simulink model "lab06es02_e1"  (R2021a)
settings: Solver=VariableStepAuto  StartTime=0.0  StopTime=150  RelTol=1e-3
values from neighbouring files (symbols this model uses):
  Kc = Kr/(Kf*0.2)    [L_11_05_21_reti_anticipatrici.m]    (also in L_11_05_21_reti_anticipatrici_2.m; L_12_05_21_Esercizio_progetto_di_un_controllore.m = 1/(0.04*Kf1*Kf2); L_12_05_21_effetti_sul_comando.m = 4; L_12_05_21_reti_integro-derivative.m = 4)
  Kr = 1    [L_11_05_21_reti_anticipatrici.m]    (also in L_11_05_21_reti_anticipatrici_2.m; L_12_05_21_Esercizio_progetto_di_un_controllore.m; L_12_05_21_effetti_sul_comando.m; L_12_05_21_reti_integro-derivative.m)
libraries: cstblocks x1, simulink x1
settings Model: Creator=fornasierarmando  LastModifiedBy=fornasierarmando

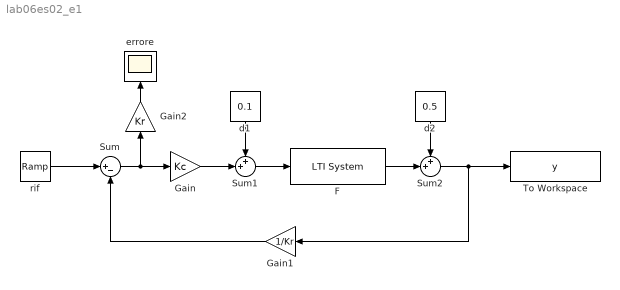
== system lab06es02_e1 ==
  F : cstblocks/LTI System  sys=F  IC=[]
  Gain : Gain  Gain=Kc
  Gain1 : Gain  Gain=1/Kr
  Gain2 : Gain  Gain=Kr
  Sum : Sum  Inputs=|+-
  Sum1 : Sum  Inputs=++|
  Sum2 : Sum  Inputs=++|
  To Workspace : ToWorkspace  VariableName=y  SaveFormat=Timeseries  SampleTime=-1
  d1 : Constant  Value=0.1
  d2 : Constant  Value=0.5
  errore : Scope
  rif : simulink/Sources/Ramp  slope=1  start=0  InitialOutput=0
  wires:
  Gain1/1 -> Sum/2
  rif/1 -> Sum/1
  Gain/1 -> Sum1/2
  Sum/1 -> Gain2/1, Gain/1
  d2/1 -> Sum2/1
  Gain2/1 -> errore/1
  d1/1 -> Sum1/1
  Sum1/1 -> F/1
  Sum2/1 -> To Workspace/1, Gain1/1
  F/1 -> Sum2/2
